simulink model "model"  (R2025b)
settings: Solver=ode4  StartTime=0.0  StopTime=20  FixedStep=0.01  RelTol=1e-3
InitFcn:
  | setup;
values from neighbouring files (symbols this model uses):
  K_GAIN = 1.0    (= 1)    [setup.m]
  N = 1000    [plot_data.m]    (also in setup.m)
  P_GAIN = 50.0    (= 50)    [setup.m]
  phase_offsets = [PHASE_OFFSET_RAD(1), -PHASE_OFFSET_RAD(1)]    [setup.m]
  robot_params = struct()    [setup.m]
undefined symbols (not defined in the file or in its folder): tables1, tables2, X, Y, Z
libraries: sm_lib x15, nesl_utility x9
settings Model: Creator=mahdi  LastModifiedBy=root
settings SolverCC: AlgebraicLoopSolver=TrustRegion
settings DebuggingCC: UnconnectedInputMsg=warning  UnconnectedOutputMsg=warning  UnconnectedLineMsg=warning
settings ModelReferenceCC: EnableRefExpFcnMdlSchedulingChecks=on
settings RTWCC: GPUComputeCapability=3.5  DLArmComputeVersion=19.05

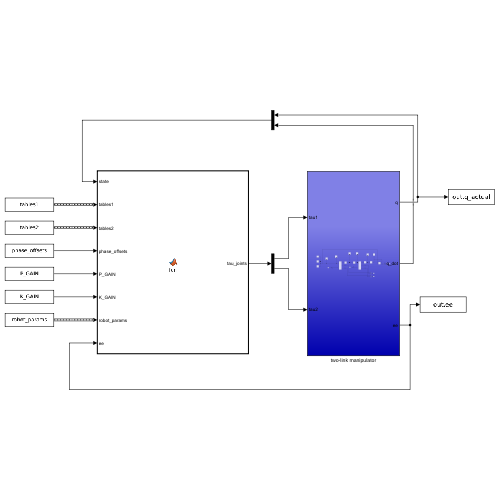
[thumbnail: Simulink's stored preview of the top-level diagram]
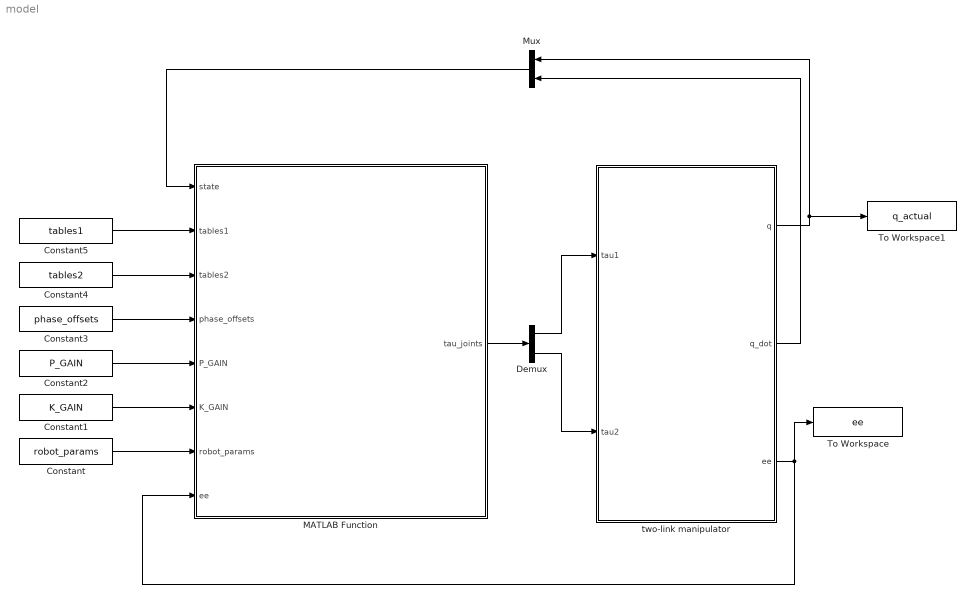
== system model ==
  Constant : Constant  Value=robot_params  OutDataTypeStr=Bus: bus_RobotParams
  Constant1 : Constant  Value=K_GAIN
  Constant2 : Constant  Value=P_GAIN
  Constant3 : Constant  Value=phase_offsets
  Constant4 : Constant  Value=tables2  OutDataTypeStr=Bus: bus_Table
  Constant5 : Constant  Value=tables1  OutDataTypeStr=Bus:bus_Table
  Demux : Demux  Outputs=2
  MATLAB Function : MATLAB Function  TreatAsAtomicUnit=on
  Mux : Mux  Inputs=2
  To Workspace : ToWorkspace  VariableName=ee  SaveFormat=Timeseries  SampleTime=-1
  To Workspace1 : ToWorkspace  VariableName=q_actual  SaveFormat=Timeseries  SampleTime=-1
  two-link manipulator : Subsystem
  wires:
  two-link manipulator/1(q) -> Mux/1, To Workspace1/1
  two-link manipulator/3(ee) -> To Workspace/1, MATLAB Function/8(ee)
  MATLAB Function/1(tau_joints) -> Demux/1
  Demux/1 -> two-link manipulator/1(tau1)
  Demux/2 -> two-link manipulator/2(tau2)
  Constant/1 -> MATLAB Function/7(robot_params)
  Constant1/1 -> MATLAB Function/6(K_GAIN)
  Constant2/1 -> MATLAB Function/5(P_GAIN)
  Constant3/1 -> MATLAB Function/4(phase_offsets)
  Constant4/1 -> MATLAB Function/3(tables2)
  Constant5/1 -> MATLAB Function/2(tables1)
  two-link manipulator/2(q_dot) -> Mux/2
  Mux/1 -> MATLAB Function/1(state)

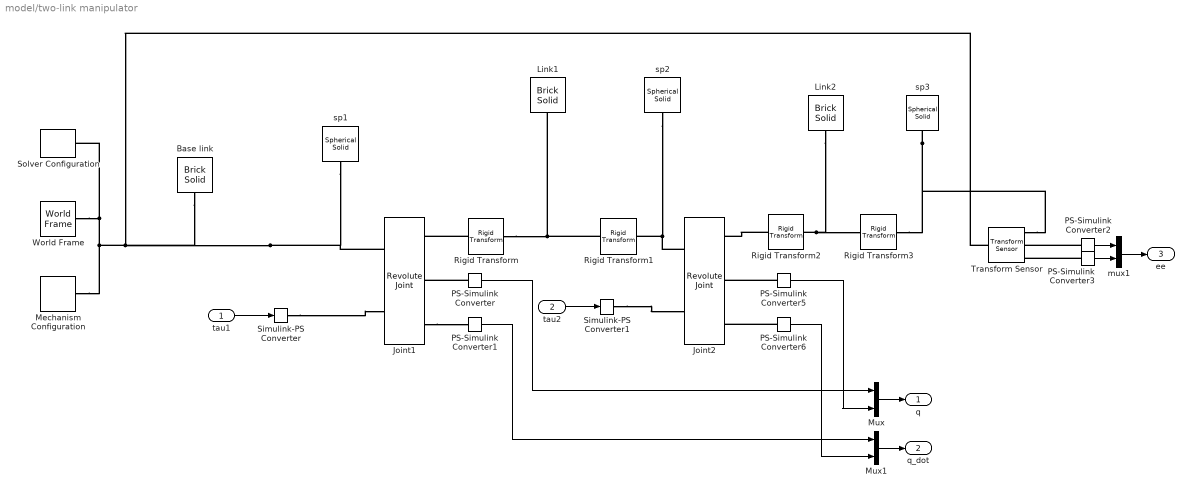
== system model/two-link manipulator ==
  tau1 : Inport
  tau2 : Inport  Port=2
  Base link : sm_lib/Body Elements/Brick Solid  BrickDimensions=[3 0.03 0.03]  BrickDimensionsUnits=m  ExportEntireGeometry=off  InertiaType=PointMass  BasedOnType=Density  Density=1000  DensityUnits=kg/m^3  Mass=0  MassUnits=kg  CenterOfMass=[0 0 0]  CenterOfMassUnits=m  MomentsOfInertia=[1 1 1]  MomentsOfInertiaUnits=kg*m^2  ProductsOfInertia=[0 0 0]  ProductsOfInertiaUnits=kg*m^2  GraphicType=FromGeometry  MarkerShape=Sphere  MarkerSize=10  GraphicVisPropType=SimpleVisualProperties  GraphicDiffuseColor=[0.2 0.0 0.2]  GraphicOpacity=1.0  GraphicSpecularColor=[0.5 0.5 0.5 1.0]  GraphicAmbientColor=[0.15 0.15 0.15 1.0]  GraphicEmissiveColor=[0.0 0.0 0.0 1.0]  GraphicShininess=75  DoExposeReferenceFrame=on  SerializedFrames=<Frames/>
  Joint1 : sm_lib/Joints/Revolute Joint  JointMode=Normal  CompositeWrenchDir=FollowerOnBase  CompositeWrenchFrame=BaseFrame  SenseConstraintForce=off  SenseConstraintTorque=off  SenseTotalForce=off  SenseTotalTorque=off  PositionTargetSpecify=on  PositionTargetPriority=High  PositionTargetValue=0.3  PositionTargetValueUnits=rad  VelocityTargetSpecify=on  VelocityTargetPriority=High  VelocityTargetValue=0  VelocityTargetValueUnits=deg/s  EquilibriumPosition=0  EquilibriumPositionUnits=deg  SpringStiffness=0  SpringStiffnessUnits=N*m/deg  DampingCoefficient=0  DampingCoefficientUnits=N*m/(deg/s)  LowerLimitSpecify=off  LowerLimitBound=-90  LowerLimitBoundUnits=deg  LowerLimitStiffness=1e4  LowerLimitStiffnessUnits=N*m/deg  LowerLimitDamping=10  LowerLimitDampingUnits=N*m/(deg/s)  LowerLimitTransitionRegionWidth=0.1  LowerLimitTransitionRegionWidthUnits=deg  UpperLimitSpecify=off  UpperLimitBound=90  UpperLimitBoundUnits=deg  UpperLimitStiffness=1e4  UpperLimitStiffnessUnits=N*m/deg  UpperLimitDamping=10  UpperLimitDampingUnits=N*m/(deg/s)  UpperLimitTransitionRegionWidth=0.1  UpperLimitTransitionRegionWidthUnits=deg  TorqueActuationMode=InputTorque  MotionActuationMode=ComputedMotion  SensePosition=on  SenseVelocity=on  SenseAcceleration=off  SenseTorqueForce=off  SenseLowerLimitTorqueForce=off  SenseUpperLimitTorqueForce=off
  Joint2 : sm_lib/Joints/Revolute Joint  JointMode=Normal  CompositeWrenchDir=FollowerOnBase  CompositeWrenchFrame=BaseFrame  SenseConstraintForce=off  SenseConstraintTorque=off  SenseTotalForce=off  SenseTotalTorque=off  PositionTargetSpecify=on  PositionTargetPriority=High  PositionTargetValue=-pi/1.7  PositionTargetValueUnits=rad  VelocityTargetSpecify=on  VelocityTargetPriority=High  VelocityTargetValue=0  VelocityTargetValueUnits=deg/s  EquilibriumPosition=0  EquilibriumPositionUnits=deg  SpringStiffness=0  SpringStiffnessUnits=N*m/deg  DampingCoefficient=0  DampingCoefficientUnits=N*m/(deg/s)  LowerLimitSpecify=off  LowerLimitBound=-90  LowerLimitBoundUnits=deg  LowerLimitStiffness=1e4  LowerLimitStiffnessUnits=N*m/deg  LowerLimitDamping=10  LowerLimitDampingUnits=N*m/(deg/s)  LowerLimitTransitionRegionWidth=0.1  LowerLimitTransitionRegionWidthUnits=deg  UpperLimitSpecify=off  UpperLimitBound=90  UpperLimitBoundUnits=deg  UpperLimitStiffness=1e4  UpperLimitStiffnessUnits=N*m/deg  UpperLimitDamping=10  UpperLimitDampingUnits=N*m/(deg/s)  UpperLimitTransitionRegionWidth=0.1  UpperLimitTransitionRegionWidthUnits=deg  TorqueActuationMode=InputTorque  MotionActuationMode=ComputedMotion  SensePosition=on  SenseVelocity=on  SenseAcceleration=off  SenseTorqueForce=off  SenseLowerLimitTorqueForce=off  SenseUpperLimitTorqueForce=off
  Link1 : sm_lib/Body Elements/Brick Solid  BrickDimensions=[1 0.1 0.1]  BrickDimensionsUnits=m  ExportEntireGeometry=off  InertiaType=CalculateFromGeometry  BasedOnType=Mass  Density=7800  DensityUnits=kg/m^3  Mass=1  MassUnits=kg  CenterOfMass=[0 0 0]  CenterOfMassUnits=m  MomentsOfInertia=[1 1 1]  MomentsOfInertiaUnits=kg*m^2  ProductsOfInertia=[0 0 0]  ProductsOfInertiaUnits=kg*m^2  GraphicType=FromGeometry  MarkerShape=Sphere  MarkerSize=10  GraphicVisPropType=SimpleVisualProperties  GraphicDiffuseColor=[0.0 0.0 0.5]  GraphicOpacity=1.0  GraphicSpecularColor=[0.5 0.5 0.5 1.0]  GraphicAmbientColor=[0.15 0.15 0.15 1.0]  GraphicEmissiveColor=[0.0 0.0 0.0 1.0]  GraphicShininess=75  DoExposeReferenceFrame=on  SerializedFrames=<Frames/>
  Link2 : sm_lib/Body Elements/Brick Solid  BrickDimensions=[1 0.1 0.1]  BrickDimensionsUnits=m  ExportEntireGeometry=off  InertiaType=CalculateFromGeometry  BasedOnType=Mass  Density=7800  DensityUnits=kg/m^3  Mass=1  MassUnits=kg  CenterOfMass=[0 0 0]  CenterOfMassUnits=m  MomentsOfInertia=[1 1 1]  MomentsOfInertiaUnits=kg*m^2  ProductsOfInertia=[0 0 0]  ProductsOfInertiaUnits=kg*m^2  GraphicType=FromGeometry  MarkerShape=Sphere  MarkerSize=10  GraphicVisPropType=SimpleVisualProperties  GraphicDiffuseColor=[0.0 0.0 0.5]  GraphicOpacity=1.0  GraphicSpecularColor=[0.5 0.5 0.5 1.0]  GraphicAmbientColor=[0.15 0.15 0.15 1.0]  GraphicEmissiveColor=[0.0 0.0 0.0 1.0]  GraphicShininess=75  DoExposeReferenceFrame=on  SerializedFrames=<Frames/>
  Mechanism Configuration : sm_lib/Utilities/Mechanism Configuration  UniformGravity=Constant  GravityVector=[0 -9.81 0]  GravityVectorUnits=m/s^2  LinearizationDelta=0.001  JointModeTransitionNonlinearIterations=2
  Mux : Mux  Inputs=2
  Mux1 : Mux  Inputs=2
  PS-Simulink Converter{,1..3,5..6} (6 alike) : nesl_utility/PS-Simulink Converter  PhysicalDomain=network_engine_domain  SubClassName=ps_output  LeftPortType=input  RightPortType=output  PseudoPeriodic=off  Frequencies=[]  VectorFormat=1-D array  Unit=inherit  AffineConversion=off
  Rigid Transform{,1..3} (4 alike) : sm_lib/Frames and Transforms/Rigid Transform  RotationMethod=None  FollAlignAxisA=+X  BaseAlignAxisA=+Y  FollAlignAxisB=+Y  BaseAlignAxisB=+Z  RotationStandardAxis=+Z  RotationAngle=0.0  RotationAngleUnits=deg  RotationArbitraryAxis=[0 0 1]  RotationSequenceAxes=FollowerAxes  RotationSequence=XYX  RotationSequenceAngles=[0 0 0]  RotationSequenceAnglesUnits=deg  RotationMatrix=[1 0 0; 0 1 0; 0 0 1]  Quaternion=[1 0 0 0]  TranslationMethod=StandardAxis  TranslationCartesianOffset=[0 0 0]  TranslationCartesianOffsetUnits=m  TranslationStandardAxis=+X  TranslationStandardOffset=0.5  TranslationStandardOffsetUnits=m  TranslationROffset=0  TranslationROffsetUnits=m  TranslationThetaOffset=0  TranslationThetaOffsetUnits=deg  TranslationZOffset=0  TranslationZOffsetUnits=m
  Simulink-PS Converter : nesl_utility/Simulink-PS Converter  PhysicalDomain=network_engine_domain  SubClassName=ps_input  LeftPortType=input  RightPortType=output  PseudoPeriodic=off  Frequencies=[]  NoiseDistribution=none  NoiseParameters=[]  Unit=1  AffineConversion=off  FilteringAndDerivatives=provide  SimscapeFilterOrder=1  InputFilterTimeConstant=0.001  UdotUserProvided=0
  Simulink-PS Converter1 : nesl_utility/Simulink-PS Converter  PhysicalDomain=network_engine_domain  SubClassName=ps_input  LeftPortType=input  RightPortType=output  PseudoPeriodic=off  Frequencies=[]  NoiseDistribution=none  NoiseParameters=[]  Unit=1  AffineConversion=off  FilteringAndDerivatives=provide  SimscapeFilterOrder=1  InputFilterTimeConstant=0.001  UdotUserProvided=0
  Solver Configuration : nesl_utility/Solver Configuration  PhysicalDomain=network_engine_domain  SubClassName=solver  LeftPortType=input  RightPortType=generic  Tones=[]  Harmonics=[]  SimulateNoise=off  Profile=off  UseLocalSampling=off  EnableSwitchedLinearOptims=on  FrequencyDomain=off  UseCCode=off  RelTol=0.001  AbsTol=1e-06  MinStep=1e-09  ToWorkspace=off  RevertToSquareIcSolve=off  NumHomotopyIterations=100  PhasorMode=off  PhasorModeNumHarmonics=1  ConsistencySolver=NEWTON_FTOL  IndexReductionMethod=DerivativeReplacement  DoDC=off  ResidualTolerance=1e-09  ConsistencyTolSource=GLOBAL  ConsistencyAbsTol=0.001  ConsistencyRelTol=0.001  ConsistencyTolFactor=0.001  UseLocalSolver=off  LocalSolverChoice=NE_BACKWARD_EULER_ADVANCER  ResolveIndetEquations=on  FunctionEvalNumThread=1  LocalSolverSampleTime=0.001  DoFixedCost=off  MaxNonlinIter=3  MaxModeIter=2  ComputeImpulses=off  ImpulseIterations=2  LinearAlgebra=Sparse  LinearAlgebraNumThread=0  EquationFormulation=NE_TIME_EF  DelaysMemoryBudget=1024  AutomaticFiltering=on  FilteringTimeConstant=0.001  PartitionStorageMethod=AS_NEEDED  PartitionMemoryBudget=1024  PartitionMethod=FAST  MultibodyUseLocalSolver=off  MultibodyLocalSolverChoice=ODE1  MultibodyLocalSolverSampleTime=0.001
  Transform Sensor : sm_lib/Frames and Transforms/Transform Sensor  MeasurementFrame=World  RotationSequence=XYX  SenseAngle=off  SenseAxis=off  SenseQ=off  SenseR=off  SenseRotationSequence=off  SenseOmegaX=off  SenseOmegaY=off  SenseOmegaZ=off  SenseOmega=off  SenseQDot=off  SenseRDot=off  SenseRotationSequenceDot=off  SenseAlphaX=off  SenseAlphaY=off  SenseAlphaZ=off  SenseAlpha=off  SenseQDDot=off  SenseRDDot=off  SenseX=on  SenseY=on  SenseZ=off  SenseXYZ=off  SenseRad=off  SenseAzim=off  SenseDist=off  SenseInc=off  SenseXDot=off  SenseYDot=off  SenseZDot=off  SenseXYZDot=off  SenseRadDot=off  SenseAzimDot=off  SenseDistDot=off  SenseIncDot=off  SenseXDDot=off  SenseYDDot=off  SenseZDDot=off  SenseXYZDDot=off  SenseRadDDot=off  SenseAzimDDot=off  SenseDistDDot=off  SenseIncDDot=off
  World Frame : sm_lib/Frames and Transforms/World Frame
  mux1 : Mux  Inputs=2
  sp1 : sm_lib/Body Elements/Spherical Solid  SphereRadius=0.08  SphereRadiusUnits=m  ExportEntireGeometry=off  InertiaType=PointMass  BasedOnType=Density  Density=1000  DensityUnits=kg/m^3  Mass=0  MassUnits=kg  CenterOfMass=[0 0 0]  CenterOfMassUnits=m  MomentsOfInertia=[1 1 1]  MomentsOfInertiaUnits=kg*m^2  ProductsOfInertia=[0 0 0]  ProductsOfInertiaUnits=kg*m^2  GraphicType=FromGeometry  MarkerShape=Sphere  MarkerSize=10  GraphicVisPropType=SimpleVisualProperties  GraphicDiffuseColor=[0.9 0.0 0.0]  GraphicOpacity=1.0  GraphicSpecularColor=[0.5 0.5 0.5 1.0]  GraphicAmbientColor=[0.15 0.15 0.15 1.0]  GraphicEmissiveColor=[0.0 0.0 0.0 1.0]  GraphicShininess=75  DoExposeReferenceFrame=on  SerializedFrames=<Frames/>
  sp2 : sm_lib/Body Elements/Spherical Solid  SphereRadius=0.08  SphereRadiusUnits=m  ExportEntireGeometry=off  InertiaType=PointMass  BasedOnType=Density  Density=1000  DensityUnits=kg/m^3  Mass=0  MassUnits=kg  CenterOfMass=[0 0 0]  CenterOfMassUnits=m  MomentsOfInertia=[1 1 1]  MomentsOfInertiaUnits=kg*m^2  ProductsOfInertia=[0 0 0]  ProductsOfInertiaUnits=kg*m^2  GraphicType=FromGeometry  MarkerShape=Sphere  MarkerSize=10  GraphicVisPropType=SimpleVisualProperties  GraphicDiffuseColor=[0.9 0.0 0.0]  GraphicOpacity=1.0  GraphicSpecularColor=[0.5 0.5 0.5 1.0]  GraphicAmbientColor=[0.15 0.15 0.15 1.0]  GraphicEmissiveColor=[0.0 0.0 0.0 1.0]  GraphicShininess=75  DoExposeReferenceFrame=on  SerializedFrames=<Frames/>
  sp3 : sm_lib/Body Elements/Spherical Solid  SphereRadius=0.08  SphereRadiusUnits=m  ExportEntireGeometry=off  InertiaType=PointMass  BasedOnType=Density  Density=1000  DensityUnits=kg/m^3  Mass=0  MassUnits=kg  CenterOfMass=[0 0 0]  CenterOfMassUnits=m  MomentsOfInertia=[1 1 1]  MomentsOfInertiaUnits=kg*m^2  ProductsOfInertia=[0 0 0]  ProductsOfInertiaUnits=kg*m^2  GraphicType=FromGeometry  MarkerShape=Sphere  MarkerSize=10  GraphicVisPropType=SimpleVisualProperties  GraphicDiffuseColor=[0.2 1.0 0.2]  GraphicOpacity=1.0  GraphicSpecularColor=[0.5 0.5 0.5 1.0]  GraphicAmbientColor=[0.15 0.15 0.15 1.0]  GraphicEmissiveColor=[0.0 0.0 0.0 1.0]  GraphicShininess=75  DoExposeReferenceFrame=on  SerializedFrames=<Frames/>
  q : Outport
  q_dot : Outport  Port=2
  ee : Outport  Port=3
  wires:
  mux1/1 -> ee/1
  PS-Simulink Converter3/1 -> mux1/2
  PS-Simulink Converter2/1 -> mux1/1
  tau1/1 -> Simulink-PS Converter/1
  PS-Simulink Converter/1 -> Mux/1
  PS-Simulink Converter1/1 -> Mux1/1
  Mux/1 -> q/1
  Mux1/1 -> q_dot/1
  tau2/1 -> Simulink-PS Converter1/1
  PS-Simulink Converter5/1 -> Mux/2
  PS-Simulink Converter6/1 -> Mux1/2
  connections:
  PS-Simulink Converter3/LConn1 -- Transform Sensor/RConn3
  PS-Simulink Converter2/LConn1 -- Transform Sensor/RConn2
  Rigid Transform/LConn1 -- Joint1/RConn1
  Simulink-PS Converter1/RConn1 -- Joint2/LConn2
  Simulink-PS Converter/RConn1 -- Joint1/LConn2
  Rigid Transform2/LConn1 -- Joint2/RConn1
  sp3/RConn1 -- Transform Sensor/RConn1 -- Rigid Transform3/RConn1
  sp2/RConn1 -- Joint2/LConn1 -- Rigid Transform1/RConn1
  Mechanism Configuration/RConn1 -- Base link/RConn1 -- sp1/RConn1 -- Joint1/LConn1 -- Transform Sensor/LConn1 -- World Frame/RConn1 -- Solver Configuration/RConn1
  Rigid Transform2/RConn1 -- Link2/RConn1 -- Rigid Transform3/LConn1
  Rigid Transform1/LConn1 -- Link1/RConn1 -- Rigid Transform/RConn1
  PS-Simulink Converter/LConn1 -- Joint1/RConn2
  Joint1/RConn3 -- PS-Simulink Converter1/LConn1
  PS-Simulink Converter6/LConn1 -- Joint2/RConn3
  PS-Simulink Converter5/LConn1 -- Joint2/RConn2

== matlab function model/MATLAB Function ==
  data: state input; tau_joints output; tables1 input; tables2 input; phase_offsets input; P_GAIN input; K_GAIN input; robot_params input; ee input
function tau_joints = fcn(state, tables1, tables2, phase_offsets, P_GAIN, K_GAIN, robot_params, ee)
    % Extract joint and Cartesian states
    q = state(1:2);
    qdot = state(3:4);
    x = ee(1);
    y = ee(2);
    
    % Compute kinematics and Jacobian matrices
    J = get_jacob(q(1), q(2), robot_params);
    Jdot = get_jacob_dot(q(1), q(2), qdot, robot_params);
    
    vel_cart = J * qdot;
    x_axis_state = [x, vel_cart(1)];
    y_axis_state = [y, vel_cart(2)];
    
    % Determine phase angles (pitch) for each axis
    x_pitch = get_pitch(x_axis_state, tables1);
    y_pitch = get_pitch(y_axis_state, tables2);

    % Compute Virtual Energy Regulator (VER) control inputs
    xddot_ver = get_desired_acceleration(x_axis_state, y_pitch, phase_offsets(1), tables1, P_GAIN, K_GAIN);  
    yddot_ver = get_desired_acceleration(y_axis_state, x_pitch, phase_offsets(2), tables2, P_GAIN, K_GAIN); 
    F_ver = [xddot_ver; yddot_ver];
    
    % Retrieve distributed mass dynamics matrices
    [M, CG] = compute_distributed_mass_dynamics(q, qdot, robot_params);
    
    % Formulate constraint dynamics equations [M -J'; J 0] * [qddot; F] = [-CG; -Jdot*qdot + F_ver]
    coef_matrix = [M, -J'; J, zeros(2, 2)];
    b_matrix = [-CG; (-Jdot * qdot + F_ver)];
    
    % Solve for joint accelerations and constraint forces (Fx, Fy)
    results = coef_matrix \ b_matrix;
    
    % Map constraint forces back to joint torques
    tau_joints = J' * [results(3); results(4)];
end

function u_ver = get_desired_acceleration(current_state, other_joint_pitch, phase_offset_rad, table, P, K)
    % Shift coordinate system to table center
    x_centered = current_state(1) - table.center;
    x_dot = current_state(2);
    
    current_theta = atan2(x_dot, x_centered);
    current_r_sq = x_centered^2 + x_dot^2;

    % Wrap theta to match the table's definition range
    min_theta = table.theta(1);
    max_theta = table.theta(end);
    current_theta_interp = min_theta + mod(current_theta - min_theta, max_theta - min_theta);

    % Interpolate reference radius and damping term
    desired_r_d = interp1(table.theta, table.r_d, current_theta_interp, 'linear');
    beta = interp1(table.theta, table.beta, current_theta_interp, 'linear');
    
    current_pitch = get_pitch(current_state, table); 

    % Calculate control components: energy regulation (alpha) and phase synchronization (gamma)
    alpha = P * tanh(x_dot) * (desired_r_d^2 - current_r_sq);
    gamma = K * (sin(other_joint_pitch + phase_offset_rad) - sin(current_pitch));

    u_ver = alpha + beta + gamma;
end

function current_pitch = get_pitch(current_state, table)
    % Direct phase mapping relative to the center
    current_theta = atan2(current_state(2), current_state(1) - table.center);
    
    if isnan(current_theta)
        current_theta = 0;
    end
            
    current_pitch = current_theta;
end

function [M, CG] = compute_distributed_mass_dynamics(q, q_dot, ~)
    % Note: Magic numbers (101/600, 981/200) indicate non-parametric hardcoding.
    q1 = q(1); q2 = q(2);
    dq1 = q_dot(1); dq2 = q_dot(2);
  
    % Inertia Matrix components
    m11 = ((sin(q1 + q2) + 2*sin(q1))*(sin(q1 + q2)/2 + sin(q1)))/2 + cos(q1)^2/4 + sin(q1)^2/4 + ((cos(q1 + q2) + 2*cos(q1))*(cos(q1 + q2)/2 + cos(q1)))/2 + 101/600;
    m12 = (cos(q1 + q2)*(cos(q1 + q2)/2 + cos(q1)))/2 + (sin(q1 + q2)*(sin(q1 + q2)/2 + sin(q1)))/2 + 101/1200;
    m22 = cos(q1 + q2)^2/4 + sin(q1 + q2)^2/4 + 101/1200;
    M = [m11, m12; m12, m22];

    % Coriolis and Gravity components
    cg1 = (981*cos(q1 + q2))/200 + (2943*cos(q1))/200 - ((2*dq1^2*sin(q1) + sin(q1 + q2)*(dq1 + dq2)^2)*(cos(q1 + q2)/2 + cos(q1)))/2 + ((sin(q1 + q2)/2 + sin(q1))*(cos(q1 + q2)*(dq1 + dq2)^2 + 2*dq1^2*cos(q1)))/2;
    cg2 = (981*cos(q1 + q2))/200 - (cos(q1 + q2)*(dq1^2*sin(q1) + (sin(q1 + q2)*(dq1 + dq2)^2)/2))/2 + (sin(q1 + q2)*((cos(q1 + q2)*(dq1 + dq2)^2)/2 + dq1^2*cos(q1)))/2;
    CG = [cg1; cg2];
end

function [M, CG] = compute_point_mass_dynamics(q, q_dot, params)
    q1 = q(1); q2 = q(2); 
    q1_dot = q_dot(1); q2_dot = q_dot(2);
    
    % Inertia Matrix
    M11 = (params.m1 + params.m2)*params.L1^2 + params.m2*params.L2^2 + 2*params.m2*params.L1*params.L2*cos(q2);
    M12 = params.m2*params.L2^2 + params.m2*params.L1*params.L2*cos(q2);
    M22 = params.m2*params.L2^2;
    M = [M11, M12; M12, M22];
     
    % Coriolis Matrix
    C11 = -params.m2*params.L1*params.L2*sin(q2)*q2_dot;
    C12 = -params.m2*params.L1*params.L2*sin(q2)*(q1_dot + q2_dot);
    C21 =  params.m2*params.L1*params.L2*sin(q2)*q1_dot;
    C = [C11, C12; C21, 0];
     
    % Gravity Vector
    g12 = -(params.m1+params.m2)*params.g*params.L1*sin(q1) - params.m2*params.g*params.L2*sin(q1+q2);
    g21 = -params.m2*params.L2*params.g*sin(q1 + q2);
    G = [g12; g21];
    
    CG = C*q_dot + G;
end

function [x, y] = forward_kinematics(q1, q2, params)
    x = params.L1 * cos(q1) + params.L2 * cos(q1 + q2);
    y = params.L1 * sin(q1) + params.L2 * sin(q1 + q2);
end

function J = get_jacob(q1, q2, params)
    s1 = sin(q1); c1 = cos(q1);
    s12 = sin(q1 + q2); c12 = cos(q1 + q2);
    
    J = [-params.L1*s1 - params.L2*s12, -params.L2*s12;
          params.L1*c1 + params.L2*c12,  params.L2*c12];
end
    
function Jdot = get_jacob_dot(q1, q2, q_dot, params)
    dq_sum = q_dot(1) + q_dot(2);
    
    c1 = cos(q1); s1 = sin(q1);
    c12 = cos(q1 + q2); s12 = sin(q1 + q2);
    
    Jdot_11 = -params.L1*c1*q_dot(1) - params.L2*c12*dq_sum;
    Jdot_12 = -params.L2*c12*dq_sum;
    Jdot_21 = -params.L1*s1*q_dot(1) - params.L2*s12*dq_sum;
    Jdot_22 = -params.L2*s12*dq_sum;
    
    Jdot = [Jdot_11, Jdot_12; Jdot_21, Jdot_22];
end
